simulink model "Scenario_13_CoDeSys"  (R2012b)
settings: Solver=ode3  StartTime=0.0  StopTime=inf  FixedStep=Sample_Time_Model  RelTol=1e-3
PreLoadFcn:
  | Variablen_Scenario13
InitFcn:
  | BT = randperm(9);
values from neighbouring files (symbols this model uses):
  Band_Geschwindigkeit = 1.47    [Variablen_Scenario13.m]
  Band_Sensor_Hell_2_Z = -6.5    [Variablen_Scenario13.m]
  Band_Sensor_Hell_3_Z = -10.36    [Variablen_Scenario13.m]
  Band_Sensor_Hell_4_Z = -14.64    [Variablen_Scenario13.m]
  Band_Sensor_Tolerance_Z = 0.2    [Variablen_Scenario13.m]
  Bauteil_Fallgeschwindigkeit = 0.4    [Variablen_Scenario13.m]
  Bauteil_Farbe_Metall = [0.8 0.8 0.8]    [Variablen_Scenario13.m]
  Bauteil_Farbe_Schwarz = [0.2 0.2 0.2]    [Variablen_Scenario13.m]
  Bauteil_Farbe_Weiss = [1 1 0.2]    [Variablen_Scenario13.m]
  Kran_Dauer_90_Grad = 5    [Variablen_Scenario13.m]
  Kran_Drehwinkel_90_Grad = 8050    [Variablen_Scenario13.m]
  Kran_Sensor_Position_Delta = 0.07    [Variablen_Scenario13.m]
  Sample_Time_Model = 0.05    [Variablen_Scenario13.m]
  Sample_Time_Simulation = 0.1    [Variablen_Scenario13.m]
  Sensor_Band_Metall_1 = -6.5    [Variablen_Scenario13.m]
  Sensor_Band_Metall_2 = -10.36    [Variablen_Scenario13.m]
libraries: simulink x557, vrlib x13, opclib x7, rtwinlib x1
(part 1 of 10)
settings Model: Creator=Aicher  LastModifiedBy=Aicher
settings DataIOCC: SignalLoggingSaveFormat=ModelDataLogs
settings OptimizationCC: EfficientMapNaN2IntZero=off
settings DebuggingCC: MultiTaskDSMMsg=warning  MultiTaskCondExecSysMsg=none  StrictBusMsg=None
settings HardwareCC: TargetIntDivRoundTo=Zero  TargetEndianess=LittleEndian  TargetHWDeviceType=MATLAB Host  ProdEqTarget=off
settings CodeAppCC: MaxIdLength=128
settings GRTTargetCC: CombineOutputUpdateFcns=off  GRTInterface=on

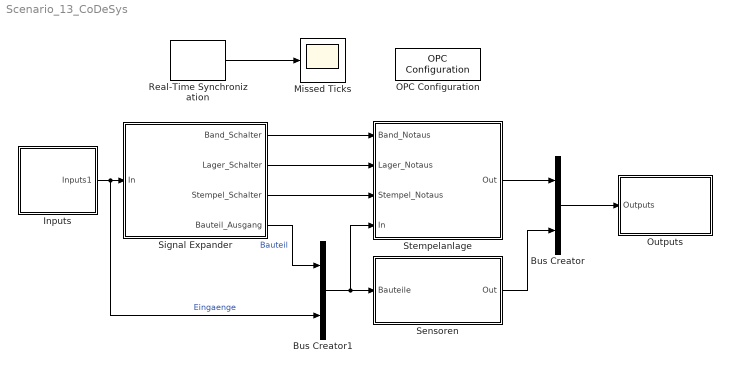
== system Scenario_13_CoDeSys ==
  Bus Creator : BusCreator  Inputs=2
  Bus Creator1 : BusCreator  Inputs=2
  Inputs : Subsystem
  Missed Ticks : Scope
      settings: TimeRange=45  YMin=0  YMax=1  DataFormat=Structure
  OPC Configuration : opclib/OPC Configuration  opcServers=localhost/CoDeSys.OPC.DA/10  errMissingItems=Error  errReadWrite=Warn  errShutdown=Error  errRTViolation=Warn  rtEnable=off  speedup=1  showLatency=off  beingUsed=on
  Outputs : Subsystem
  Real-Time Synchronization : rtwinlib/Real-Time Synchronization  SampleTime=Sample_Time_Model  MaxMissedTicks=100  ShowMissedTicks=on  YieldWhenWaiting=off
  Sensoren : Subsystem
  Signal Expander : Subsystem
  Stempelanlage : Subsystem
  wires:
  Inputs/1(Inputs1) -> Bus Creator1/2, Signal Expander/1(In)  "Eingaenge"
  Signal Expander/4(Bauteil_Ausgang) -> Bus Creator1/1  "Bauteil"
  Signal Expander/2(Lager_Schalter) -> Stempelanlage/2(Lager_Notaus)
  Stempelanlage/1(Out) -> Bus Creator/1
  Sensoren/1(Out) -> Bus Creator/2
  Bus Creator/1 -> Outputs/1(Outputs)
  Bus Creator1/1 -> Stempelanlage/4(In), Sensoren/1(Bauteile)
  Real-Time Synchronization/1 -> Missed Ticks/1
  Signal Expander/1(Band_Schalter) -> Stempelanlage/1(Band_Notaus)
  Signal Expander/3(Stempel_Schalter) -> Stempelanlage/3(Stempel_Notaus)

== system Scenario_13_CoDeSys/Inputs ==
  Bus Creator10 : BusCreator  Inputs=5
  Bus Creator11 : BusCreator  Inputs=9
  Bus Creator6 : BusCreator  Inputs=6
  Bus Creator7 : BusCreator  Inputs=6
  Bus Creator8 : BusCreator  Inputs=7
  Bus Creator9 : BusCreator  Inputs=3
  Demux2 : Demux  Outputs=19
  Demux3 : Demux  Outputs=3
  OPC Read2 : opclib/OPC Read  serverHost=localhost  serverID=CoDeSys.OPC.DA  itemIDs=PLC_GW3.Application.GVL.Stempel_Druck_Soll, PLC_GW3.Application.GVL.Stempelschlitten.QX_einfahren, PLC_GW3.Application.GVL.Stempelschlitten.QX_ausfahren, PLC_GW3.Application.GVL.Stempelzylinder.QX_einfahren, PLC_GW3.Application.GVL.Stempelzylinder.QX_ausfahren, PLC_GW3.Application.GVL.Band_vor, PLC_GW3.Application.GVL.Band_zurueck, PLC_GW3.Application.GVL.Sortierzylinder1.QX_einfahren, PLC_GW3.Application.GVL.Sortierzylinder1.QX_ausfahren, PLC_GW3.Application.GVL.Sortierzylinder2.QX_einfahren, PLC_GW3.Application.GVL.Sortierzylinder2.QX_ausfahren, PLC_GW3.Application.GVL.Vereinzelungszylinder.QX_einfahren, PLC_GW3.Application.GVL.Vereinzelungszylinder.QX_ausfahren, PLC_GW3.Application.GVL.Kran_Sauger_an, PLC_GW3.Application.GVL.Kran_Sauger_aus, PLC_GW3.Application.GVL.Kran_drehen_links, PLC_GW3.Application.GVL.Kran_drehen_rechts, PLC_GW3.Application.GVL.Kranzylinder.QX_einfahren, PLC_GW3.Application.GVL.Kranzylinder.QX_ausfahren  readMode=Asynchronous (device)  dataType=double  updateRate=Sample_Time_OPC_Fast  showQual=off  showTS=off  tsMode=Seconds since start
  OPC Read3 : opclib/OPC Read  serverHost=localhost  serverID=CoDeSys.OPC.DA  itemIDs=PLC_GW3.Application.GVL.Lager_Lampe_Gruen, PLC_GW3.Application.GVL.Band_Lampe_Gruen, PLC_GW3.Application.GVL.Stempel_Lampe_Gruen  readMode=Asynchronous (device)  dataType=double  updateRate=Sample_Time_OPC_Fast  showQual=off  showTS=off  tsMode=Seconds since start
  Rate Transition2 : RateTransition
  Rate Transition3 : RateTransition
  Subsystem1 : Subsystem
  Inputs1 : Outport
  wires:
  Demux2/15 -> Bus Creator6/2  "Kran_Sauger_Aus"
  Demux2/13 -> Bus Creator9/3  "Lager_Zyl_ausfahren"
  Demux2/12 -> Bus Creator9/2  "Lager_Zyl_einfahren"
  Demux2/11 -> Bus Creator8/7  "Band_Zyl_2_ausfahren"
  Demux2/9 -> Bus Creator8/5  "Band_Zyl_1_ausfahren"
  Demux2/10 -> Bus Creator8/6  "Band_Zyl_2_einfahren"
  Demux2/7 -> Bus Creator8/3  "Band_zurueck"
  Demux2/8 -> Bus Creator8/4  "Band_Zyl_1_einfahren"
  Demux2/5 -> Bus Creator7/6  "Stempel_ausfahren"
  Demux2/6 -> Bus Creator8/2  "Band_vor"
  Demux2/3 -> Bus Creator7/4  "Stempel_Halterung_ausfahren"
  Demux2/2 -> Bus Creator7/3  "Stempel_Halterung_einfahren"
  Demux2/4 -> Bus Creator7/5  "Stempel_einfahren"
  Bus Creator6/1 -> Bus Creator10/5  "Kran"
  Bus Creator7/1 -> Bus Creator10/2  "Stempel"
  Bus Creator8/1 -> Bus Creator10/3  "Band"
  Bus Creator9/1 -> Bus Creator10/4  "Lager"
  Bus Creator10/1 -> Inputs1/1  "Inputs"
  Subsystem1/1(BT1) -> Bus Creator11/1  "BT_Eins"
  Subsystem1/2(BT2) -> Bus Creator11/2  "BT_Zwei"
  Subsystem1/3(BT3) -> Bus Creator11/3  "BT_Drei"
  Subsystem1/4(BT4) -> Bus Creator11/4  "BT_Vier"
  Subsystem1/5(BT5) -> Bus Creator11/5  "BT_Fuenf"
  Subsystem1/6(BT6) -> Bus Creator11/6  "BT_Sechs"
  Bus Creator11/1 -> Bus Creator10/1  "Bauteile"
  OPC Read2/1 -> Rate Transition2/1
  Demux2/14 -> Bus Creator6/1  "Kran_Sauger_An"
  OPC Read3/1 -> Rate Transition3/1
  Demux2/16 -> Bus Creator6/3  "Kran_Drehen_Links"
  Demux2/17 -> Bus Creator6/4  "Kran_Drehen_Rechts"
  Demux2/18 -> Bus Creator6/5  "Kran_einfahren"
  Demux2/19 -> Bus Creator6/6  "Kran_ausfahren"
  Rate Transition3/1 -> Demux3/1
  Rate Transition2/1 -> Demux2/1
  Demux3/2 -> Bus Creator8/1  "Band_Lampe_Gruen"
  Demux2/1 -> Bus Creator7/2  "Stempel_Druck_Soll"
  Demux3/3 -> Bus Creator7/1  "Stempel_Lampe_Gruen"
  Demux3/1 -> Bus Creator9/1  "Lager_Lampe_Gruen"
  Subsystem1/7(BT7) -> Bus Creator11/7  "BT_Sieben"
  Subsystem1/8(BT8) -> Bus Creator11/8  "BT_Acht"
  Subsystem1/9(BT9) -> Bus Creator11/9  "BT_Neun"

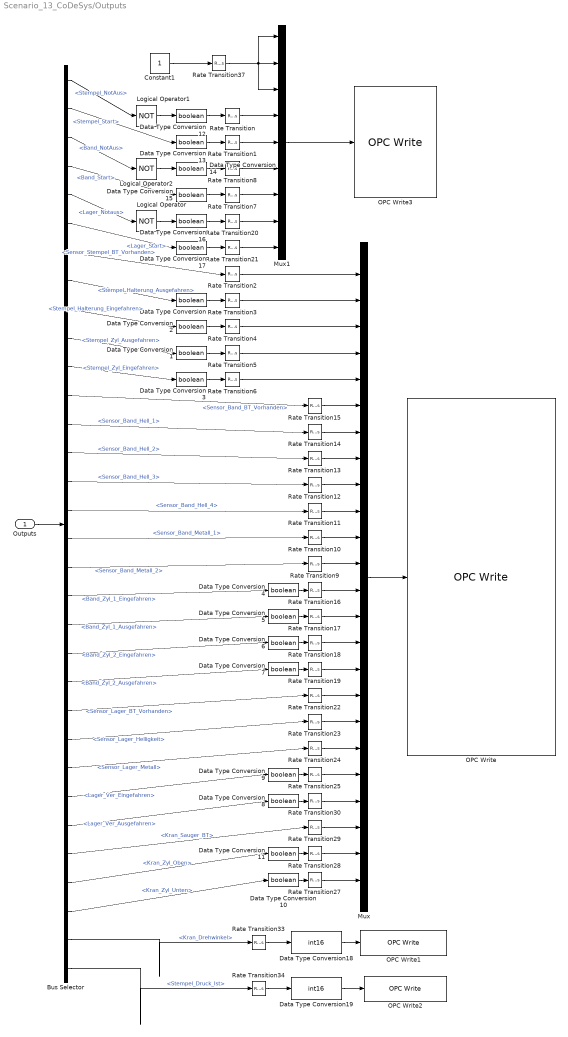
== system Scenario_13_CoDeSys/Outputs ==
  Outputs : Inport
  Bus Selector : BusSelector  OutputSignals=signal1.Stempel_Schalter.Stempel_NotAus,signal1.Stempel_Schalter.Stempel_Start,signal1.Band_Schalter.Band_NotAus,signal1.Band_Schalter.Band_Start,signal1.Lager_Schalter.Lager_Notaus,signal1.Lager_Schalter.Lager_Start,Sensoren.Sensor_Stempel_BT_Vorhanden,signal1.signal1.Bauteil.Stempelanlage_BT.Stempelanlage.Stempel.Stempel_Halterung_Ausgefahren,signal1.signal1.Bauteil.Stempelanlage_BT.Stempelanlage.Stempel.Stempel_Halterung_Eingefahren,signal1.signal1.Bauteil.Stempelanlage_BT.Stempelanlage.Stempel.Stempel_Zyl.Stempel_Zyl_Ausgefahren,signal1.signal1.Bauteil.Stempelanlage_BT.Stempelanlage.Stempel.Stempel_Zyl.Stempel_Zyl_Eingefahren,Sensoren.Sensor_Band_BT_Vorhanden,Sensoren.Sensor_Band_Hell_1,Sensoren.Sensor_Band_Hell_2,Sensoren.Sensor_Band_Hell_3,Sensoren.Sensor_Band_Hell_4,Sensoren.Sensor_Band_Metall_1,Sensoren.Sensor_Band_Metall_2,signal1.signal1.Bauteil.Stempelanlage_BT.Stempelanlage.Band.Band_Zyl_1_Eingefahren,signal1.signal1.Bauteil.Stempelanlage_BT.Stempelanlage.Band.Band_Zyl_1_Ausgefahren,signal1.signal1.Bauteil.Stempelanlage_BT.Stempelanlage.Band.Band_Zyl_2_Eingefahren,signal1.signal1.Bauteil.Stempelanlage_BT.Stempelanlage.Band.Band_Zyl_2_Ausgefahren,Sensoren.Sensor_Lager_BT_Vorhanden,Sensoren.Sensor_Lager_Helligkeit,Sensoren.Sensor_Lager_Metall,signal1.signal1.Bauteil.Stempelanlage_BT.Stempelanlage.Lager.Lager_Ver_Eingefahren,signal1.signal1.Bauteil.Stempelanlage_BT.Stempelanlage.Lager.Lager_Ver_Ausgefahren,Sensoren.Kran_Sauger_BT,signal1.signal1.Bauteil.Stempelanlage_BT.Stempelanlage.Kran.Kran_Zyl.Kran_Zyl_Oben,signal1.signal1.Bauteil.Stempelanlage_BT.Stempelanlage.Kran.Kran_Zyl.Kran_Zyl_Unten,signal1.signal1.Bauteil.Stempelanlage_BT.Stempelanlage.Kran.Kran_Drehwinkel,Sensoren.Stempel_Druck_Ist
  Constant1 : Constant  OutDataTypeStr=boolean
  Data Type Conversion{,1..17} (18 alike) : DataTypeConversion  OutDataTypeStr=boolean
  Data Type Conversion18 : DataTypeConversion  OutDataTypeStr=int16
  Data Type Conversion19 : DataTypeConversion  OutDataTypeStr=int16
  Logical Operator : Logic  Operator=NOT  AllPortsSameDT=off  OutDataTypeStr=boolean
  Logical Operator1 : Logic  Operator=NOT  AllPortsSameDT=off
  Logical Operator2 : Logic  Operator=NOT  AllPortsSameDT=off  OutDataTypeStr=boolean
  Mux : Mux  Inputs=24
  Mux1 : Mux  Inputs=9
  OPC Write : opclib/OPC Write  serverHost=localhost  serverID=CoDeSys.OPC.DA  itemIDs=PLC_GW3.Application.GVL.Stempel_Sensor_Mat_vorhanden, PLC_GW3.Application.GVL.Stempelschlitten.IX_ausgefahren, PLC_GW3.Application.GVL.Stempelschlitten.IX_eingefahren, PLC_GW3.Application.GVL.Stempelzylinder.IX_ausgefahren, PLC_GW3.Application.GVL.Stempelzylinder.IX_eingefahren, PLC_GW3.Application.GVL.Band_Sensor_Mat_Vorhanden, PLC_GW3.Application.GVL.Band_Sensor_Hell_1, PLC_GW3.Application.GVL.Band_Sensor_Hell_2, PLC_GW3.Application.GVL.Band_Sensor_Hell_3, PLC_GW3.Application.GVL.Band_Sensor_Hell_4, PLC_GW3.Application.GVL.Band_Sensor_Metall_1, PLC_GW3.Application.GVL.Band_Sensor_Metall_2, PLC_GW3.Application.GVL.Sortierzylinder1.IX_eingefahren, PLC_GW3.Application.GVL.Sortierzylinder1.IX_ausgefahren, PLC_GW3.Application.GVL.Sortierzylinder2.IX_eingefahren, PLC_GW3.Application.GVL.Sortierzylinder2.IX_ausgefahren, PLC_GW3.Application.GVL.Lager_Sensor_Mat_Vorhanden, PLC_GW3.Application.GVL.Lager_Sensor_Hell, PLC_GW3.Application.GVL.Lager_Sensor_Metall, PLC_GW3.Application.GVL.Vereinzelungszylinder.IX_eingefahren, PLC_GW3.Application.GVL.Vereinzelungszylinder.IX_ausgefahren, PLC_GW3.Application.GVL.Kran_Mat_angesaugt, PLC_GW3.Application.GVL.Kranzylinder.IX_ausgefahren, PLC_GW3.Application.GVL.Kranzylinder.IX_eingefahren  writeMode=Asynchronous  updateRate=0.1
  OPC Write1 : opclib/OPC Write  serverHost=localhost  serverID=CoDeSys.OPC.DA  itemIDs=PLC_GW3.Application.GVL.Kran_Drehwinkel  writeMode=Asynchronous  updateRate=0.05
  OPC Write2 : opclib/OPC Write  serverHost=localhost  serverID=CoDeSys.OPC.DA  itemIDs=PLC_GW3.Application.GVL.Stempel_Druck_Ist  writeMode=Asynchronous  updateRate=0.1
  OPC Write3 : opclib/OPC Write  serverHost=localhost  serverID=CoDeSys.OPC.DA  itemIDs=PLC_GW3.Application.GVL.Stempel_Man_Auto, PLC_GW3.Application.GVL.Band_Man_Auto, PLC_GW3.Application.GVL.Lager_Man_Auto, PLC_GW3.Application.GVL.Nicht_Notaus_Stempel, PLC_GW3.Application.GVL.Stempel_Start, PLC_GW3.Application.GVL.Nicht_Notaus_Band, PLC_GW3.Application.GVL.Band_Start, PLC_GW3.Application.GVL.Nicht_Notaus_Lager, PLC_GW3.Application.GVL.Lager_Start  writeMode=Asynchronous  updateRate=0.1
  Rate Transition{,1..25,27..30,33..34,37} (33 alike) : RateTransition
  wires:
  Outputs/1 -> Bus Selector/1
  Bus Selector/30 -> Data Type Conversion10/1  "<Kran_Zyl_Unten>"
  Bus Selector/5 -> Logical Operator/1  "<Lager_Notaus>"
  Bus Selector/19 -> Data Type Conversion4/1  "<Band_Zyl_1_Eingefahren>"
  Bus Selector/8 -> Data Type Conversion/1  "<Stempel_Halterung_Ausgefahren>"
  Bus Selector/11 -> Data Type Conversion3/1  "<Stempel_Zyl_Eingefahren>"
  Bus Selector/23 -> Rate Transition22/1  "<Sensor_Lager_BT_Vorhanden>"
  Bus Selector/1 -> Logical Operator1/1  "<Stempel_NotAus>"
  Bus Selector/21 -> Data Type Conversion6/1  "<Band_Zyl_2_Eingefahren>"
  Bus Selector/3 -> Logical Operator2/1  "<Band_NotAus>"
  Bus Selector/9 -> Data Type Conversion2/1  "<Stempel_Halterung_Eingefahren>"
  Bus Selector/6 -> Data Type Conversion17/1  "<Lager_Start>"
  Bus Selector/7 -> Rate Transition2/1  "<Sensor_Stempel_BT_Vorhanden>"
  Bus Selector/22 -> Data Type Conversion7/1  "<Band_Zyl_2_Ausgefahren>"
  Bus Selector/10 -> Data Type Conversion1/1  "<Stempel_Zyl_Ausgefahren>"
  Bus Selector/20 -> Data Type Conversion5/1  "<Band_Zyl_1_Ausgefahren>"
  Bus Selector/2 -> Data Type Conversion13/1  "<Stempel_Start>"
  Bus Selector/24 -> Rate Transition23/1  "<Sensor_Lager_Helligkeit>"
  Bus Selector/27 -> Data Type Conversion8/1  "<Lager_Ver_Ausgefahren>"
  Bus Selector/25 -> Rate Transition24/1  "<Sensor_Lager_Metall>"
  Bus Selector/26 -> Data Type Conversion9/1  "<Lager_Ver_Eingefahren>"
  Bus Selector/29 -> Data Type Conversion11/1  "<Kran_Zyl_Oben>"
  Bus Selector/28 -> Rate Transition29/1  "<Kran_Sauger_BT>"
  Mux/1 -> OPC Write/1
  Data Type Conversion/1 -> Rate Transition3/1
  Data Type Conversion2/1 -> Rate Transition4/1
  Data Type Conversion1/1 -> Rate Transition5/1
  Data Type Conversion3/1 -> Rate Transition6/1
  Data Type Conversion4/1 -> Rate Transition16/1
  Data Type Conversion5/1 -> Rate Transition17/1
  Data Type Conversion7/1 -> Rate Transition19/1
  Data Type Conversion9/1 -> Rate Transition25/1
  Data Type Conversion8/1 -> Rate Transition30/1
  Data Type Conversion11/1 -> Rate Transition28/1
  Data Type Conversion10/1 -> Rate Transition27/1
  Bus Selector/31 -> Rate Transition33/1  "<Kran_Drehwinkel>"
  Bus Selector/4 -> Data Type Conversion15/1  "<Band_Start>"
  Bus Selector/32 -> Rate Transition34/1  "<Stempel_Druck_Ist>"
  Data Type Conversion6/1 -> Rate Transition18/1
  Logical Operator/1 -> Data Type Conversion16/1
  Logical Operator1/1 -> Data Type Conversion12/1
  Logical Operator2/1 -> Data Type Conversion14/1
  Constant1/1 -> Rate Transition37/1
  Mux1/1 -> OPC Write3/1
  Rate Transition/1 -> Mux1/4
  Rate Transition1/1 -> Mux1/5
  Rate Transition2/1 -> Mux/1
  Rate Transition3/1 -> Mux/2
  Rate Transition4/1 -> Mux/3
  Rate Transition5/1 -> Mux/4
  Rate Transition6/1 -> Mux/5
  Rate Transition8/1 -> Mux1/6
  Rate Transition7/1 -> Mux1/7
  Rate Transition16/1 -> Mux/13
  Rate Transition17/1 -> Mux/14
  Rate Transition18/1 -> Mux/15
  Rate Transition19/1 -> Mux/16
  Rate Transition20/1 -> Mux1/8
  Rate Transition21/1 -> Mux1/9
  Rate Transition22/1 -> Mux/17
  Rate Transition23/1 -> Mux/18
  Rate Transition24/1 -> Mux/19
  Rate Transition25/1 -> Mux/20
  Rate Transition30/1 -> Mux/21
  Rate Transition29/1 -> Mux/22
  Rate Transition28/1 -> Mux/23
  Rate Transition27/1 -> Mux/24
  Rate Transition33/1 -> Data Type Conversion18/1
  Rate Transition34/1 -> Data Type Conversion19/1
  Rate Transition37/1 -> Mux1/3, Mux1/1, Mux1/2
  Data Type Conversion12/1 -> Rate Transition/1
  Data Type Conversion17/1 -> Rate Transition21/1
  Data Type Conversion16/1 -> Rate Transition20/1
  Data Type Conversion15/1 -> Rate Transition7/1
  Data Type Conversion14/1 -> Rate Transition8/1
  Data Type Conversion13/1 -> Rate Transition1/1
  Bus Selector/13 -> Rate Transition14/1  "<Sensor_Band_Hell_1>"
  Bus Selector/18 -> Rate Transition9/1  "<Sensor_Band_Metall_2>"
  Bus Selector/17 -> Rate Transition10/1  "<Sensor_Band_Metall_1>"
  Bus Selector/16 -> Rate Transition11/1  "<Sensor_Band_Hell_4>"
  Bus Selector/15 -> Rate Transition12/1  "<Sensor_Band_Hell_3>"
  Bus Selector/14 -> Rate Transition13/1  "<Sensor_Band_Hell_2>"
  Bus Selector/12 -> Rate Transition15/1  "<Sensor_Band_BT_Vorhanden>"
  Rate Transition9/1 -> Mux/12
  Rate Transition10/1 -> Mux/11
  Rate Transition11/1 -> Mux/10
  Rate Transition12/1 -> Mux/9
  Rate Transition13/1 -> Mux/8
  Rate Transition14/1 -> Mux/7
  Rate Transition15/1 -> Mux/6
  Data Type Conversion18/1 -> OPC Write1/1
  Data Type Conversion19/1 -> OPC Write2/1

== system Scenario_13_CoDeSys/Sensoren ==
  Bauteile : Inport
  Bus Creator1 : BusCreator  Inputs=13
  Bus Selector4 : BusSelector  OutputSignals=Bauteil.Stempelanlage_BT.Bauteil_1.Kran_Sauger_BT_1,Bauteil.Stempelanlage_BT.Bauteil_2.Kran_Sauger_BT_2,Bauteil.Stempelanlage_BT.Bauteil_3.Kran_Sauger_BT_3,Bauteil.Stempelanlage_BT.Bauteil_4.Kran_Sauger_BT_4,Bauteil.Stempelanlage_BT.Bauteil_5.Kran_Sauger_BT_5,Bauteil.Stempelanlage_BT.Bauteil_6.Kran_Sauger_BT_6,Bauteil.Stempelanlage_BT.Bauteil_7.Kran_Sauger_BT_7,Bauteil.Stempelanlage_BT.Bauteil_8.Kran_Sauger_BT_8,Bauteil.Stempelanlage_BT.Bauteil_9.Kran_Sauger_BT_9
  Bus Selector5 : BusSelector  OutputSignals=Bauteil.Stempelanlage_BT.Stempelanlage.Stempel.Stempel_Halterung_Eingefahren,Bauteil.Stempelanlage_BT.Stempelanlage.Stempel.Stempel_Zyl.Stempel_Zyl_Ausgefahren
  Bus Selector6 : BusSelector  OutputSignals=Eingaenge.Stempel.Stempel_Druck_Soll
  Display{,1..12} (13 alike) : Display
  Kran_Sauger_BT : Subsystem
  Sensor_Band_BT_Vorhanden_Hell_1 : Subsystem
  Sensor_Band_Hell_2 : Subsystem
  Sensor_Band_Hell_3 : Subsystem
  Sensor_Band_Hell_4 : Subsystem
  Sensor_Band_Metall_1 : Subsystem
  Sensor_Band_Metall_2 : Subsystem
  Sensor_Lager_BT_Vorhanden : Subsystem
  Sensor_Stempel_BT_Vorhanden : Subsystem
  Sensoren_Lager_Metall_und_Weiss_Schwarz : Subsystem
  Stempel_Druck_Ist : Subsystem
  Out : Outport
  wires:
  Bus Selector4/1 -> Kran_Sauger_BT/1(BT_1)  "<Kran_Sauger_BT_1>"
  Bus Selector4/2 -> Kran_Sauger_BT/2(BT_2)  "<Kran_Sauger_BT_2>"
  Sensor_Stempel_BT_Vorhanden/1(Sensor_Stempel_BT_Vorhanden) -> Stempel_Druck_Ist/1(Sensor_Stempel_BT_Vorhanden), Display/1, Bus Creator1/5  "Sensor_Stempel_BT_Vorhanden"
  Kran_Sauger_BT/1(Kran_Sauger_BT) -> Display1/1, Bus Creator1/4  "Kran_Sauger_BT"
  Sensor_Lager_BT_Vorhanden/1(Sensor_Lager_BT_Vorhanden) -> Display2/1, Bus Creator1/3  "Sensor_Lager_BT_Vorhanden"
  Bus Creator1/1 -> Out/1  "Sensoren"
  Bus Selector5/1 -> Stempel_Druck_Ist/2(Stempel_Halterung_Eingefahren)  "<Stempel_Halterung_Eingefahren>"
  Bus Selector5/2 -> Stempel_Druck_Ist/3(Stempel_Zyl_Ausgefahren)  "<Stempel_Zyl_Ausgefahren>"
  Stempel_Druck_Ist/1(Stempel_Druck_Ist) -> Display5/1, Bus Creator1/6  "Stempel_Druck_Ist"
  Bus Selector6/1 -> Stempel_Druck_Ist/4(Stempel_Druck_Soll)  "<Stempel_Druck_Soll>"
  Sensoren_Lager_Metall_und_Weiss_Schwarz/1(Sensor_Lager_Metall) -> Display4/1, Bus Creator1/1  "Sensor_Lager_Metall"
  Sensoren_Lager_Metall_und_Weiss_Schwarz/2(Sensor_Lager_Helligkeit) -> Display3/1, Bus Creator1/2  "Sensor_Lager_Helligkeit"
  Bauteile/1 -> Sensoren_Lager_Metall_und_Weiss_Schwarz/1(In), Sensor_Lager_BT_Vorhanden/1(In), Sensor_Band_Hell_4/1(Inputs), Sensor_Band_Metall_2/1(Inputs), Sensor_Band_Metall_1/1(Inputs), Sensor_Band_Hell_3/1(Inputs), Sensor_Band_Hell_2/1(Inputs), Sensor_Band_BT_Vorhanden_Hell_1/1(Inputs), Bus Selector6/1, Bus Selector5/1, Sensor_Stempel_BT_Vorhanden/1(In), Bus Selector4/1
  Bus Selector4/3 -> Kran_Sauger_BT/3(BT_3)  "<Kran_Sauger_BT_3>"
  Bus Selector4/6 -> Kran_Sauger_BT/6(BT_6)  "<Kran_Sauger_BT_6>"
  Bus Selector4/5 -> Kran_Sauger_BT/5(BT_5)  "<Kran_Sauger_BT_5>"
  Bus Selector4/4 -> Kran_Sauger_BT/4(BT_4)  "<Kran_Sauger_BT_4>"
  Bus Selector4/7 -> Kran_Sauger_BT/7(BT_7)  "<Kran_Sauger_BT_7>"
  Bus Selector4/9 -> Kran_Sauger_BT/9(BT_9)  "<Kran_Sauger_BT_9>"
  Bus Selector4/8 -> Kran_Sauger_BT/8(BT_8)  "<Kran_Sauger_BT_8>"
  Sensor_Band_BT_Vorhanden_Hell_1/1(Sensor_Band_BT_Vorhanden) -> Display6/1, Bus Creator1/7  "Sensor_Band_BT_Vorhanden"
  Sensor_Band_BT_Vorhanden_Hell_1/2(Sensor_Band_Hell_1) -> Display7/1, Bus Creator1/8  "Sensor_Band_Hell_1"
  Sensor_Band_Hell_2/1(Sensor_Band_Hell_2) -> Display8/1, Bus Creator1/9  "Sensor_Band_Hell_2"
  Sensor_Band_Hell_4/1(Sensor_Band_Hell_4) -> Display10/1, Bus Creator1/11  "Sensor_Band_Hell_4"
  Sensor_Band_Metall_1/1(Sensor_Band_Metall_1) -> Display11/1, Bus Creator1/12  "Sensor_Band_Metall_1"
  Sensor_Band_Metall_2/1(Sensor_Band_Metall_2) -> Bus Creator1/13, Display12/1  "Sensor_Band_Metall_2"
  Sensor_Band_Hell_3/1(Sensor_Band_Hell_3) -> Display9/1, Bus Creator1/10  "Sensor_Band_Hell_3"

== stateflow chart Scenario_13_CoDeSys/Signal Expander/Bauteil_7 ==
  state Bauteil_Pos_7
    entry:
    BT_X_Achse = 5.75;
    BT_Y_Achse = 6.84;
    x =0;
  state Bauteil_Faellt3
    during:
    BT_Y_Achse = Next_Pos_Minus_Min(BT_Y_Achse, Bauteil_Fallgeschwindigkeit, 5.83);
  state Bauteil_Pos_6
    entry:
    BT_X_Achse = 5.75;
    BT_Y_Achse = 5.81;
    x =0;
  state Bauteil_Faellt2
    during:
    BT_Y_Achse = Next_Pos_Minus_Min(BT_Y_Achse, Bauteil_Fallgeschwindigkeit, 4.8);
  state Stop1
  state Bauteil_Pos_2
  state Bauteil_Unten
  state Bauteil_Pos_5
  state Bauteil_Faellt_3
    during:
    BT_Y_Achse = Next_Pos_Minus_Min(BT_Y_Achse, Bauteil_Fallgeschwindigkeit, 0.7);
  state Drehen_Rechts_Runter [function]
    (default) -> (junction 322) : {BT_Y_Achse = Next_Pos_Minus_Min(BT_Y_Achse, Kran_Zyl_Schritt_Runter, 0.65);
        | x = x - Kran_Drehen_Schritt;
        | BT_Z_Achse = -3.5*sin(x);
        | BT_X_Achse = 3.5*cos(x);}
  state Bauteil_Faellt1
    during:
    BT_Y_Achse = Next_Pos_Minus_Min(BT_Y_Achse, Bauteil_Fallgeschwindigkeit, 3.77);
  state Drehen_Rechts_Hoch [function]
    (default) -> (junction 325) : {BT_Y_Achse = Next_Pos_Plus_Max(BT_Y_Achse, Kran_Zyl_Schritt_Hoch, 1.65);
        | x = x - Kran_Drehen_Schritt;
        | BT_Z_Achse = -3.5*sin(x);
        | BT_X_Achse = 3.5*cos(x);}
  state Bauteil_Lager_Vereinz_Ausfahren
    during:
    BT_X_Achse = BT_X_Achse - Lager_Vereinzler_Schritt_Aus;
  state Bauteil_Lager_Bereit
    entry: BT_Bereit = 1;
    BT_X_Achse = 3.5;
  state Drehen_Links_Runter [function]
    (default) -> (junction 319) : {BT_Y_Achse = Next_Pos_Minus_Min(BT_Y_Achse, Kran_Zyl_Schritt_Runter, 0.65);
        | x = x + Kran_Drehen_Schritt;
        | BT_Z_Achse = -3.5*sin(x);
        | BT_X_Achse = 3.5*cos(x);}
  state Drehen_Links_Hoch [function]
    (default) -> (junction 309) : {BT_Y_Achse = Next_Pos_Plus_Max(BT_Y_Achse, Kran_Zyl_Schritt_Hoch, 1.65);
        | x = x + Kran_Drehen_Schritt;
        | BT_Z_Achse = -3.5*sin(x);
        | BT_X_Achse = 3.5*cos(x);}
  state Ausgabe = Next_Pos_Plus_Max(Achse, Schrittgroesse, MaxWert) [function]
    (default) -> (junction 249) : {Naechste_Position = Achse + Schrittgroesse;}
    (junction 249) -> (junction 250) [order 1] : [Naechste_Position >= MaxWert]
    (junction 249) -> (junction 251) [order 2] : {Ausgabe = Naechste_Position;}
    (junction 250) -> (junction 252) : {Ausgabe = MaxWert;}
    (junction 252) -> (junction 251)
  state Bauteil_Pos_3
  state Bauteil_Kran_Hochheben_Bereit
    entry: BT_Bereit = 1;
    Kran_Sauger_BT = 1;
  state Bauteil_Faellt_2
    during:
    BT_Y_Achse = Next_Pos_Minus_Min(BT_Y_Achse, Bauteil_Fallgeschwindigkeit, 1.73);
  state Bauteil_Pos_4
  state Bauteil_Faellt
    during:
    BT_Y_Achse = Next_Pos_Minus_Min(BT_Y_Achse, Bauteil_Fallgeschwindigkeit, 2.75);
  state Ausgabe = Next_Pos_Minus_Min(Achse, Schrittgroesse, MinWert) [function]
    (default) -> (junction 268) : {Naechste_Position = Achse - Schrittgroesse;}
    (junction 268) -> (junction 269) [order 1] : [Naechste_Position <= MinWert]
    (junction 268) -> (junction 270) [order 2] : {Ausgabe = Naechste_Position;}
    (junction 269) -> (junction 271) : {Ausgabe = MinWert;}
    (junction 271) -> (junction 270)
  state Ausgabe = Lager_Y_Achse(Lager_Status, Pos_1, Pos_2, Pos_3) [function]
    (default) -> (junction 398)
    (junction 398) -> (junction 397) [order 3] : [Lager_Status == 2]
    (junction 398) -> (junction 399) [order 1] : [Lager_Status == 0]
    (junction 397) -> (junction 400) : {Ausgabe = Pos_3;}
    (junction 398) -> (junction 401) [order 2] : [Lager_Status == 1]
        | {Ausgabe = Pos_2;}
    (junction 399) -> (junction 402) : {Ausgabe = Pos_1;}
    (junction 400) -> (junction 401)
    (junction 402) -> (junction 401)
  state Bauteil_Stempel_Halterung_Einfahren
    during:
    BT_X_Achse = Next_Pos_Minus_Min(BT_X_Achse, Stempel_Halterung_Schritt_Ein, -4.6);
  state Bauteil_Kran_Runterlassen
    during:
    BT_Y_Achse = Next_Pos_Minus_Min(BT_Y_Achse, Kran_Zyl_Schritt_Runter, 0.65);
  state Bauteil_Kran_Hochheben
    during:
    BT_Y_Achse = Next_Pos_Plus_Max(BT_Y_Achse, Kran_Zyl_Schritt_Hoch, 1.65);
  state Bauteil_Faellt_Auf_Festen_Untergrund
  state Bauteil_Lost
  state Bauteil_Lager_1_Ende
    entry: BT_Y_Achse = Lager_Y_Achse(Lager_1_Status, -0.158, 0.037, 0.232);
    BT_Lager = 1;
  state Bauteil_Abgesetzt_Stempel
    entry: Kran_Sauger_BT = 0;
  state Bauteil_Kran_Zyl_Stop
  state Bauteil_Stempel_Halterung_Stop
  state Drop_Down
    entry: Kran_Sauger_BT = 0;
    during:
    BT_Y_Achse = BT_Y_Achse - 0.4;
  state Bauteil_Lager_1_Beginnt
    entry: BT_Rotation_1 = 0;
    BT_Rotation_2 = 0;
    BT_Rotation_3 = 1;
    BT_Rotation_4 = 0.2;
    during:
    BT_X_Achse = Next_Pos_Minus_Min(BT_X_Achse, Band_Zyl_1_Schritt, -6.5 + Lager_1_Status);
    BT_Y_Achse = BT_Y_Achse - (0.2 * Band_Zyl_1_Schritt);
  state Bauteil_Stempel_Halterung_Ausfahren
    during:
    BT_X_Achse = Next_Pos_Plus_Max(BT_X_Achse, Stempel_Halterung_Schritt_Aus, -3.4);
  note: Bei -2,8 beginnt in etwa die Schraege !!
  state Drehen_Links
    during:
    x = x + Kran_Drehen_Schritt;
    BT_Z_Achse = -3.5*sin(x);
    BT_X_Achse = 3.5*cos(x);
  state Bauteil_Band_Vor
    during:
    BT_Z_Achse = BT_Z_Achse - Band_Geschwindigkeit;
  state Bauteil_Lager_1_Schieben
    during:
    BT_X_Achse = Next_Pos_Minus_Min(BT_X_Achse, Band_Zyl_1_Schritt, -2.7);
  state Bauteil_Lager_2_Ende
    entry: BT_Y_Achse = Lager_Y_Achse(Lager_2_Status, -0.158, 0.037, 0.232);
    BT_Lager = 2;
  state Bauteil_Kran_Rot_Stop
  state Bauteil_Band_Stop
    entry: Kran_Sauger_BT = 0;
  state Drehen_Rechts
    during:
    x = x - Kran_Drehen_Schritt;
    BT_Z_Achse = -3.5*sin(x);
    BT_X_Achse = 3.5*cos(x);
  state Bauteil_Lager_2_Beginnt
    entry: BT_Rotation_1 = 0;
    BT_Rotation_2 = 0;
    BT_Rotation_3 = 1;
    BT_Rotation_4 = 0.2;
    during:
    BT_X_Achse = Next_Pos_Minus_Min(BT_X_Achse, Band_Zyl_2_Schritt, -6.5 + Lager_2_Status);
    BT_Y_Achse = BT_Y_Achse - (0.2 * Band_Zyl_2_Schritt);
  state Bauteil_Band_Zurueck
    during:
    BT_Z_Achse = BT_Z_Achse + Band_Geschwindigkeit;
  state Bauteil_Lager_2_Schieben
    during:
    BT_X_Achse = Next_Pos_Minus_Min(BT_X_Achse, Band_Zyl_2_Schritt, -2.7);
  state Bauteil_Kran_Runterlassen_Und_Drehen_Rechts
    entry:
    x = x - Kran_Drehen_Schritt;
    BT_Z_Achse = -3.5*sin(x);
    BT_X_Achse = 3.5*cos(x);
    during: Drehen_Rechts_Runter();
  state Bauteil_Lager_3_Beginnt
    entry: BT_Rotation_1 = -1;
    BT_Rotation_2 = 0;
    BT_Rotation_3 = 0;
    BT_Rotation_4 = 0.2;
    during:
    BT_Z_Achse = Next_Pos_Minus_Min(BT_Z_Achse, 1.5 * Band_Geschwindigkeit, -19.05 + Lager_3_Status);
    BT_Y_Achse = BT_Y_Achse - (1.5 * 0.2*Band_Geschwindigkeit);
  state Bauteil_Kran_Hochheben_Und_Drehen_Links
    entry:
    x = x + Kran_Drehen_Schritt;
    BT_Z_Achse = -3.5*sin(x);
    BT_X_Achse = 3.5*cos(x);
    during: Drehen_Links_Hoch();
  state Bauteil_Lager_3_Ende
    entry: BT_Y_Achse = Lager_Y_Achse(Lager_3_Status, -0.158, 0.037, 0.232);
    BT_Lager = 3;
  state Bauteil_Kran_Hochheben_Und_Drehen_Rechts
    entry:
    x = x - Kran_Drehen_Schritt;
    BT_Z_Achse = -3.5*sin(x);
    BT_X_Achse = 3.5*cos(x);
    during:Drehen_Rechts_Hoch();
  state Bauteil_Kran_Runterlassen_Und_Drehen_Links
    entry:
    x = x + Kran_Drehen_Schritt;
    BT_Z_Achse = -3.5*sin(x);
    BT_X_Achse = 3.5*cos(x);
    during: Drehen_Links_Runter();
  (default) -> Bauteil_Pos_7
  Bauteil_Faellt_Auf_Festen_Untergrund -> Bauteil_Abgesetzt_Stempel [order 2] : [Kran_Stellung_Stempel]
  Bauteil_Pos_7 -> Bauteil_Faellt3 : [BT_1_Bereit && Lager_Ver_Eingefahren]
  Bauteil_Faellt3 -> Bauteil_Pos_6 : [BT_Y_Achse <= 5.83]
  Bauteil_Pos_6 -> Bauteil_Faellt2 : [BT_2_Bereit && Lager_Ver_Eingefahren]
  Bauteil_Faellt2 -> Bauteil_Pos_5 : [BT_Y_Achse <= 4.8]
  Stop1 -> Bauteil_Lager_Vereinz_Ausfahren : [BT_X_Achse + Lager_X_Achse >= 5.1]
  Bauteil_Lager_Vereinz_Ausfahren -> Stop1 [order 2] : [BT_X_Achse + Lager_X_Achse < 5.1]
  Bauteil_Pos_2 -> Bauteil_Faellt_3 : [BT_6_Bereit && Lager_Ver_Eingefahren]
  Bauteil_Unten -> Bauteil_Lager_Vereinz_Ausfahren : [Lager_Ver_Ausfahren && (BT_X_Achse + Lager_X_Achse >= 5.1)]
  Bauteil_Pos_5 -> Bauteil_Faellt1 : [BT_3_Bereit && Lager_Ver_Eingefahren]
  Bauteil_Faellt_2 -> Bauteil_Pos_2 : [BT_Y_Achse <= 1.73]
  Bauteil_Faellt_3 -> Bauteil_Unten : [BT_Y_Achse <= 0.7]
  Bauteil_Lager_Vereinz_Ausfahren -> Bauteil_Lager_Bereit [order 1] : [Lager_Ver_Ausgefahren]
  Bauteil_Faellt1 -> Bauteil_Pos_4 : [BT_Y_Achse <= 3.77]
  Bauteil_Faellt_Auf_Festen_Untergrund -> Bauteil_Lager_Bereit [order 1] : [Kran_Stellung_Lager]
  Bauteil_Lager_Bereit -> Bauteil_Kran_Hochheben_Bereit : [Kran_Stellung_Lager && Kran_Sauger && Kran_Zyl_Unten]
  Bauteil_Stempel_Halterung_Stop -> Bauteil_Kran_Hochheben_Bereit [order 3] : [Kran_Stellung_Stempel && Kran_Sauger && Kran_Zyl_Unten]
  (junction 127) -> Bauteil_Kran_Hochheben_Bereit [order 2] : [Kran_Stellung_Lager && Kran_Sauger && Kran_Zyl_Unten]
  Bauteil_Faellt -> Bauteil_Pos_3 : [BT_Y_Achse <= 2.75]
  Bauteil_Kran_Hochheben_Bereit -> Bauteil_Kran_Hochheben : [Kran_Hochheben]
      | {BT_Bereit = 0;}
  Bauteil_Pos_3 -> Bauteil_Faellt_2 : [BT_5_Bereit && Lager_Ver_Eingefahren]
  Bauteil_Pos_4 -> Bauteil_Faellt : [BT_4_Bereit && Lager_Ver_Eingefahren]
  Bauteil_Kran_Hochheben -> (junction 127) [order 3]
  Bauteil_Kran_Rot_Stop -> (junction 287) [order 4]
  (junction 287) -> Bauteil_Kran_Hochheben [order 2] : [Kran_Hochheben]
  (junction 287) -> Bauteil_Kran_Runterlassen [order 1] : [Kran_Runterlassen]
  Bauteil_Stempel_Halterung_Stop -> Bauteil_Stempel_Halterung_Einfahren [order 1] : [Stempel_Halterung_Einfahren]
  Bauteil_Stempel_Halterung_Einfahren -> Bauteil_Stempel_Halterung_Stop : [!Stempel_Halterung_Einfahren]
  Bauteil_Kran_Hochheben -> Bauteil_Kran_Runterlassen [order 1] : [Kran_Runterlassen]
  Bauteil_Kran_Runterlassen -> (junction 127) [order 2]
  Bauteil_Kran_Runterlassen -> (junction 162) [order 4]
  Bauteil_Kran_Zyl_Stop -> Bauteil_Kran_Runterlassen [order 3] : [Kran_Runterlassen]
  Bauteil_Kran_Runterlassen -> Bauteil_Kran_Zyl_Stop [order 3] : [Kran_Zyl_Unten]
  Bauteil_Kran_Runterlassen -> Bauteil_Kran_Hochheben [order 1] : [Kran_Hochheben]
  Drop_Down -> Bauteil_Faellt_Auf_Festen_Untergrund [order 2] : [(Kran_Stellung_Band || Kran_Stellung_Lager || Kran_Stellung_Stempel) && (BT_Y_Achse <= 0.65)]
  Drop_Down -> Bauteil_Lost [order 1] : [BT_Y_Achse <= -2]
  Bauteil_Kran_Hochheben -> (junction 162) [order 4]
  Bauteil_Kran_Hochheben -> Bauteil_Kran_Zyl_Stop [order 2] : [Kran_Zyl_Oben]
  Bauteil_Kran_Zyl_Stop -> Bauteil_Kran_Hochheben [order 2] : [Kran_Hochheben]
  Bauteil_Lager_1_Beginnt -> Bauteil_Lager_1_Ende : [BT_X_Achse <= (-6.5 + Lager_1_Status)]
  Bauteil_Abgesetzt_Stempel -> Bauteil_Stempel_Halterung_Stop
  Bauteil_Faellt_Auf_Festen_Untergrund -> Bauteil_Band_Stop [order 3] : [Kran_Stellung_Band]
  (junction 127) -> Drop_Down [order 1] : [!Kran_Sauger]
  Bauteil_Kran_Zyl_Stop -> (junction 127) [order 8]
  Bauteil_Kran_Zyl_Stop -> Bauteil_Abgesetzt_Stempel [order 6] : [Kran_Zyl_Unten && !Kran_Sauger && Kran_Stellung_Stempel]
  Drehen_Rechts -> Drop_Down [order 3] : [!Kran_Sauger]
  Bauteil_Stempel_Halterung_Ausfahren -> Bauteil_Stempel_Halterung_Stop : [!Stempel_Halterung_Ausfahren]
  Bauteil_Stempel_Halterung_Stop -> Bauteil_Stempel_Halterung_Ausfahren [order 2] : [Stempel_Halterung_Ausfahren]
  Bauteil_Kran_Rot_Stop -> Drop_Down [order 3] : [!Kran_Sauger]
  Drehen_Links -> Drop_Down [order 3] : [!Kran_Sauger]
  Bauteil_Kran_Zyl_Stop -> Drehen_Links [order 4] : [Kran_Drehen_Links]
  Bauteil_Kran_Zyl_Stop -> Drehen_Rechts [order 5] : [Kran_Drehen_Rechts]
  (junction 178) -> Bauteil_Kran_Zyl_Stop : [!Kran_Drehen_Rechts && !Kran_Drehen_Links]
  Bauteil_Kran_Zyl_Stop -> (junction 162) [order 1]
  Bauteil_Kran_Zyl_Stop -> Bauteil_Band_Stop [order 7] : [Kran_Zyl_Unten && !Kran_Sauger && Kran_Stellung_Band]
  Bauteil_Band_Stop -> Bauteil_Kran_Zyl_Stop [order 3] : [Kran_Zyl_Unten && Kran_Sauger && Kran_Stellung_Band && (-3.8 <= BT_Z_Achse) && (BT_Z_Achse <= -3.2) && (-0.3 <= BT_X_Achse) && (BT_X_Achse<= 0.3)]
  (junction 280) -> Drehen_Links [order 2] : [(Kran_Zyl_Unten || Kran_Zyl_Oben) && Kran_Drehen_Links]
      | {x = x + Kran_Drehen_Schritt;
      | BT_Z_Achse = -3.5*sin(x);
      | BT_X_Achse = 3.5*cos(x);}
  Drehen_Links -> Bauteil_Kran_Rot_Stop [order 2] : [!Kran_Drehen_Links]
  Bauteil_Lager_1_Schieben -> Bauteil_Lager_1_Beginnt : [BT_X_Achse <= -2.7]
  Bauteil_Kran_Rot_Stop -> Drehen_Links [order 1] : [Kran_Drehen_Links]
  Bauteil_Band_Vor -> (junction 135) [order 2]
  Drehen_Links -> (junction 162) [order 4]
  Drehen_Rechts -> Drehen_Links [order 1] : [Kran_Drehen_Links]
  Drehen_Links -> Drehen_Rechts [order 1] : [Kran_Drehen_Rechts]
  Bauteil_Band_Stop -> Bauteil_Band_Vor [order 1] : [Band_Vor]
  Bauteil_Band_Vor -> Bauteil_Band_Stop [order 1] : [!Band_Vor]
  (junction 135) -> Bauteil_Lager_1_Schieben [order 1] : [BT_Z_Achse <= -7.85 && BT_Z_Achse >= -8.65 && Band_Zyl_1_X_Achse >= -0.5]
  Bauteil_Lager_2_Beginnt -> Bauteil_Lager_2_Ende : [BT_X_Achse <= (-6.5 + Lager_2_Status)]
  (junction 280) -> Bauteil_Kran_Rot_Stop [order 3] : [Kran_Zyl_Unten || Kran_Zyl_Oben]
  Drehen_Rechts -> Bauteil_Kran_Rot_Stop [order 2] : [!Kran_Drehen_Rechts]
  Bauteil_Kran_Rot_Stop -> Drehen_Rechts [order 2] : [Kran_Drehen_Rechts]
  Bauteil_Band_Stop -> (junction 135) [order 4]
  (junction 135) -> Bauteil_Lager_2_Schieben [order 3] : [BT_Z_Achse <= -12.05 && BT_Z_Achse >= -12.85 && Band_Zyl_2_X_Achse >= -0.5]
  Bauteil_Band_Zurueck -> (junction 135) [order 2]
  (junction 135) -> Bauteil_Lager_3_Beginnt [order 2] : [BT_Z_Achse <= -14.6]
  Drehen_Rechts -> (junction 162) [order 4]
  Bauteil_Band_Zurueck -> Bauteil_Band_Stop [order 1] : [!Band_Zurueck]
  Bauteil_Band_Stop -> Bauteil_Band_Zurueck [order 2] : [Band_Zurueck]
  Bauteil_Kran_Runterlassen_Und_Drehen_Rechts -> (junction 178) [order 2]
  Bauteil_Kran_Hochheben_Und_Drehen_Links -> (junction 178) [order 2]
  Bauteil_Kran_Hochheben_Und_Drehen_Rechts -> (junction 178) [order 2]
  Bauteil_Kran_Runterlassen_Und_Drehen_Links -> (junction 178) [order 2]
  (junction 280) -> Drehen_Rechts [order 1] : [(Kran_Zyl_Unten || Kran_Zyl_Oben) && Kran_Drehen_Rechts]
      | {x = x - Kran_Drehen_Schritt;
      | BT_Z_Achse = -3.5*sin(x);
      | BT_X_Achse = 3.5*cos(x);}
  (junction 172) -> (junction 280)
  (junction 162) -> Bauteil_Kran_Runterlassen_Und_Drehen_Rechts [order 4] : [Kran_Drehen_Rechts && Kran_Runterlassen]
  (junction 162) -> Bauteil_Kran_Hochheben_Und_Drehen_Rechts [order 2] : [Kran_Drehen_Rechts && Kran_Hochheben]
  (junction 162) -> Bauteil_Kran_Hochheben_Und_Drehen_Links [order 1] : [Kran_Drehen_Links  && Kran_Hochheben]
  (junction 162) -> Bauteil_Kran_Runterlassen_Und_Drehen_Links [order 3] : [Kran_Drehen_Links  && Kran_Runterlassen]
  Bauteil_Lager_2_Schieben -> Bauteil_Lager_2_Beginnt : [BT_X_Achse <= -2.7]
  Bauteil_Kran_Runterlassen_Und_Drehen_Rechts -> (junction 172) [order 1]
  Bauteil_Lager_3_Beginnt -> Bauteil_Lager_3_Ende : [BT_Z_Achse <= (-19.05 + Lager_3_Status)]
  Bauteil_Kran_Hochheben_Und_Drehen_Rechts -> Bauteil_Kran_Runterlassen_Und_Drehen_Rechts [order 3] : [Kran_Drehen_Rechts  && Kran_Runterlassen]
  Bauteil_Kran_Runterlassen_Und_Drehen_Rechts -> Bauteil_Kran_Hochheben_Und_Drehen_Rechts [order 3] : [Kran_Drehen_Rechts  && Kran_Hochheben]
  Bauteil_Kran_Hochheben_Und_Drehen_Rechts -> (junction 172) [order 1]
  Bauteil_Kran_Hochheben_Und_Drehen_Links -> (junction 172) [order 1]
  Bauteil_Kran_Hochheben_Und_Drehen_Links -> Bauteil_Kran_Runterlassen_Und_Drehen_Links [order 3] : [Kran_Drehen_Links  && Kran_Runterlassen]
  Bauteil_Kran_Runterlassen_Und_Drehen_Links -> Bauteil_Kran_Hochheben_Und_Drehen_Links [order 3] : [Kran_Drehen_Links  && Kran_Hochheben]
  Bauteil_Kran_Runterlassen_Und_Drehen_Links -> (junction 172) [order 1]
  data: Achse function_input double; Schrittgroesse function_input double; MaxWert function_input double; Ausgabe function_output double; Achse function_input double; Schrittgroesse function_input double; MinWert function_input double; Ausgabe function_output double; Lager_Status function_input double; Pos_1 function_input double; Pos_2 function_input double; Ausgabe function_output double; Pos_3 function_input double; BT_Y_Achse output double; BT_Lager output double; Kran_Sauger_BT output double; BT_Bereit output double; BT_X_Achse output double; BT_Z_Achse output double; x local double; Lager_X_Achse input; Lager_Ver_Eingefahren input; Lager_Ver_Ausgefahren input; Kran_Stellung_Lager input; Kran_Stellung_Band input; Kran_Stellung_Stempel input; Kran_Zyl_Oben input; Kran_Zyl_Unten input; Kran_Sauger input; Kran_Hochheben input; Kran_Runterlassen input; Kran_Drehen_Links input; Kran_Drehen_Rechts input; Stempel_Halterung_Ausfahren input; Stempel_Halterung_Einfahren input; Band_Vor input; Band_Zurueck input; Band_Zyl_1_X_Achse input; Band_Zyl_2_X_Achse input; BT_Rotation_1 output double; BT_Rotation_2 output double; BT_Rotation_3 output double; BT_Rotation_4 output double; Lager_Ver_Ausfahren input; Lager_Vereinzler_Schritt_Aus input; Kran_Zyl_Schritt_Hoch input; Kran_Zyl_Schritt_Runter input; Kran_Drehen_Schritt input; Stempel_Halterung_Schritt_Aus input; Stempel_Halterung_Schritt_Ein input; Band_Zyl_1_Schritt input; Band_Zyl_2_Schritt input double; Band_Geschwindigkeit input; Bauteil_Fallgeschwindigkeit input double; Lager_1_Status input; Lager_2_Status input; Lager_3_Status input; Naechste_Position local double; BT_1_Bereit input; BT_2_Bereit input; BT_3_Bereit input; BT_4_Bereit input; BT_5_Bereit input; BT_6_Bereit input

== stateflow chart Scenario_13_CoDeSys/Signal Expander/Lager ==
  state r = Continue_Einfahren [function]
    (default) -> (junction 162) : {r=0}
    (junction 162) -> (junction 163) [order 1] : [Vereinzler_Einfahren && !Vereinzler_Ausfahren]
    (junction 163) -> (junction 165) : {r=1}
    (junction 162) -> (junction 164) [order 2]
    (junction 165) -> (junction 164)
  state Schrittgroesse_Ausfahren [function]
    (default) -> (junction 109) : {Schrittgroesse_Ausfahren = (1.65 * Sample_Time)/0.6}
  state Berechne_Naechste_Position_Einfahren [function]
    (default) -> (junction 118) : {Naechste_Position = Vereinzler_X_Achse - Schrittgroesse_Einfahren;}
    (junction 118) -> (junction 120) [order 1] : [Naechste_Position <= -0.65]
    (junction 118) -> (junction 122) [order 2] : {Vereinzler_X_Achse = Naechste_Position;}
    (junction 120) -> (junction 123) : {Vereinzler_X_Achse = -0.65;}
    (junction 123) -> (junction 122)
  state Schrittgroesse_Einfahren [function]
    (default) -> (junction 112) : {Schrittgroesse_Einfahren = (1.65 * Sample_Time)/0.1}
  state Berechne_Naechste_Position_Ausfahren [function]
    (default) -> (junction 208) : {Naechste_Position = Vereinzler_X_Achse + Schrittgroesse_Ausfahren;}
    (junction 208) -> (junction 209) [order 1] : [Naechste_Position >= 1.53]
    (junction 208) -> (junction 210) [order 2] : {Vereinzler_X_Achse = Naechste_Position;}
    (junction 209) -> (junction 211) : {Vereinzler_X_Achse = 1.53;}
    (junction 211) -> (junction 210)
  state r = Stop_Einfahren [function]
    (default) -> (junction 173) : {r=0}
    (junction 173) -> (junction 174) [order 1] : [!Vereinzler_Einfahren || (Vereinzler_Ausfahren && Vereinzler_Einfahren)]
    (junction 174) -> (junction 176) : {r=1}
    (junction 173) -> (junction 175) [order 2]
    (junction 176) -> (junction 175)
  state r = Continue_Ausfahren [function]
    (default) -> (junction 151) : {r=0}
    (junction 151) -> (junction 152) [order 1] : [Vereinzler_Ausfahren && !Vereinzler_Einfahren]
    (junction 152) -> (junction 154) : {r=1}
    (junction 151) -> (junction 153) [order 2]
    (junction 154) -> (junction 153)
  state Vereinzler_Bereit
    entry: Vereinzler_X_Achse = -0.65;
    Vereinzler_Eingefahren = 1;
    exit: Vereinzler_Eingefahren = 0;
  state r = Stop_Ausfahren [function]
    (default) -> (junction 184) : {r=0}
    (junction 184) -> (junction 185) [order 1] : [!Vereinzler_Ausfahren || (Vereinzler_Ausfahren && Vereinzler_Einfahren)]
    (junction 185) -> (junction 187) : {r=1}
    (junction 184) -> (junction 186) [order 2]
    (junction 187) -> (junction 186)
  state Stop1
  state Vereinzler_Ausfahren
    entry: Lager_Ver_Ausfahren = 1;
    during: Vereinzler_X_Achse = Vereinzler_X_Achse + Schrittgroesse_Ausfahren;
    exit: Lager_Ver_Ausfahren = 0;
  state Vereinzler_Ausgefahren_Fertig
    entry: Vereinzler_Ausgefahren = 1;
    Vereinzler_X_Achse = 1.6;
    exit: Vereinzler_Ausgefahren = 0;
  state Vereinzler_Einfahren
    entry: Lager_Ver_Einfahren = 1;
    during: Berechne_Naechste_Position_Einfahren();
    exit: Lager_Ver_Einfahren = 0;
  (default) -> Vereinzler_Bereit : {Schrittgroesse_Ausfahren();
      | Schrittgroesse_Einfahren()}
  Vereinzler_Bereit -> Vereinzler_Ausfahren : [Vereinzler_Ausfahren && !Vereinzler_Einfahren]
  Vereinzler_Einfahren -> Vereinzler_Bereit [order 1] : [Vereinzler_X_Achse <= -0.65]
  Vereinzler_Ausfahren -> Stop1 [order 2] : [!Stop_Einfahren()]
  Stop1 -> Vereinzler_Ausfahren [order 1] : [Continue_Ausfahren()]
  Vereinzler_Ausfahren -> Vereinzler_Ausgefahren_Fertig [order 1] : [Vereinzler_X_Achse >= 1.53]
  Stop1 -> Vereinzler_Einfahren [order 2] : [Continue_Einfahren()]
  Vereinzler_Einfahren -> Stop1 [order 2] : [Stop_Einfahren()]
  Vereinzler_Ausgefahren_Fertig -> Vereinzler_Einfahren : [Vereinzler_Einfahren && !Vereinzler_Ausfahren]
  data: r function_output double; r function_output double; r function_output double; r function_output double; Vereinzler_Einfahren input; Vereinzler_Ausfahren input; Sample_Time input; Vereinzler_X_Achse output double; Vereinzler_Eingefahren output double; Vereinzler_Ausgefahren output double; Lager_Ver_Einfahren output double; Lager_Ver_Ausfahren output double; Schrittgroesse_Ausfahren output double; Schrittgroesse_Einfahren output double; Naechste_Position local double

== stateflow chart Scenario_13_CoDeSys/Signal Expander/Halterung_Stempel ==
  state Halterung_Bereit_Ausgefahren
    entry: Halterung_X_Achse = -1.1;
    Stempel_Halterung_Ausgefahren = 1;
    exit: Stempel_Halterung_Ausgefahren = 0;
  state r = Stop_Einfahren [function]
    (default) -> (junction 63) : {r=0}
    (junction 63) -> (junction 65) [order 1] : [!Halterung_Einfahren || (Halterung_Ausfahren && Halterung_Einfahren)]
    (junction 65) -> (junction 66) : {r=1}
    (junction 63) -> (junction 64) [order 2]
    (junction 66) -> (junction 64)
  state Stop
  state r = Stop_Ausfahren [function]
    (default) -> (junction 77) : {r=0}
    (junction 77) -> (junction 78) [order 1] : [!Halterung_Ausfahren || (Halterung_Ausfahren && Halterung_Einfahren)]
    (junction 78) -> (junction 80) : {r=1}
    (junction 77) -> (junction 79) [order 2]
    (junction 80) -> (junction 79)
  state Halterung_Einfahren
    entry: Stempel_Halterung_Einfahren_FS = 1;
    during: Halterung_X_Achse = Halterung_X_Achse + Schrittgroesse_Einfahren;
    exit: Stempel_Halterung_Einfahren_FS = 0;
  state r = Continue_Einfahren [function]
    (default) -> (junction 88) : {r=0}
    (junction 88) -> (junction 89) [order 1] : [Halterung_Einfahren && !Halterung_Ausfahren]
    (junction 89) -> (junction 91) : {r=1}
    (junction 88) -> (junction 90) [order 2]
    (junction 91) -> (junction 90)
  state Halterung_Eingefahren
    entry: Stempel_Halterung_Eingefahren = 1;
    exit: Stempel_Halterung_Eingefahren = 0;
  state r = Continue_Ausfahren [function]
    (default) -> (junction 110) : {r=0}
    (junction 110) -> (junction 111) [order 1] : [Halterung_Ausfahren && !Halterung_Einfahren]
    (junction 111) -> (junction 113) : {r=1}
    (junction 110) -> (junction 112) [order 2]
    (junction 113) -> (junction 112)
  state Schrittgroesse_Ausfahren [function]
    (default) -> (junction 124) : {Schrittgroesse_Ausfahren = (1.1 * Sample_Time)/0.53}
  state Halterung_ausfahren
    entry: Stempel_Halterung_Ausfahren_FS = 1;
    during: Berechne_Naechste_Position_Ausfahren();
    exit: Stempel_Halterung_Ausfahren_FS = 0;
  state Schrittgroesse_Einfahren [function]
    (default) -> (junction 127) : {Schrittgroesse_Einfahren = (1.1 * Sample_Time)/0.56}
  state Berechne_Naechste_Position_Ausfahren [function]
    (default) -> (junction 133) : {Naechste_Position = Halterung_X_Achse - Schrittgroesse_Ausfahren;}
    (junction 133) -> (junction 134) [order 1] : [Naechste_Position <= -1.1]
    (junction 133) -> (junction 135) [order 2] : {Halterung_X_Achse = Naechste_Position;}
    (junction 134) -> (junction 136) : {Halterung_X_Achse = -1.1;}
    (junction 136) -> (junction 135)
  (default) -> Halterung_Bereit_Ausgefahren : {Schrittgroesse_Ausfahren();
      | Schrittgroesse_Einfahren()}
  Halterung_Bereit_Ausgefahren -> Halterung_Einfahren : [Halterung_Einfahren && !Halterung_Ausfahren]
  Halterung_ausfahren -> Halterung_Bereit_Ausgefahren [order 1] : [Halterung_X_Achse <= -1.1]
  Halterung_Einfahren -> Stop [order 2] : [Stop_Einfahren()]
  Stop -> Halterung_Einfahren [order 2] : [Continue_Einfahren()]
  Halterung_Einfahren -> Halterung_Eingefahren [order 1] : [Halterung_X_Achse >= 0]
  Stop -> Halterung_ausfahren [order 1] : [Continue_Ausfahren()]
  Halterung_ausfahren -> Stop [order 2] : [Stop_Ausfahren()]
  Halterung_Eingefahren -> Halterung_ausfahren : [Halterung_Ausfahren && !Halterung_Einfahren]
  data: r function_output double; r function_output double; r function_output double; r function_output double; Halterung_Ausfahren input; Halterung_Einfahren input; Halterung_X_Achse output double; Stempel_Halterung_Ausgefahren output double; Stempel_Halterung_Eingefahren output double; Stempel_Halterung_Ausfahren_FS output double; Stempel_Halterung_Einfahren_FS output double; Sample_Time input; Schrittgroesse_Ausfahren output double; Schrittgroesse_Einfahren output double; Naechste_Position local double

== stateflow chart Scenario_13_CoDeSys/Signal Expander/Kran ==
  note: 90 Grad = 1.5708
  note: KRan benoetigt fuer 90 Grad 2,6 sek
  state r = Stop_Drehen_Links [function]
    (default) -> (junction 143) : {r=0}
    (junction 143) -> (junction 144) [order 1] : [(!Kran_Drehen_Links || (Kran_Drehen_Links && Kran_Drehen_Rechts)) || (Kran_Stellung >= 3.927)]
    (junction 144) -> (junction 146) : {r=1}
    (junction 143) -> (junction 145) [order 2]
    (junction 146) -> (junction 145)
  state Kran_Drehen_Rechts
    entry: Kran_Drehen_Rechts_FS = 1;
    during: Kran_Stellung = Kran_Stellung - Schrittgroesse_Drehen;
    Kran_Drehwinkel = Kran_Drehwinkel + ((Kran_Drehwinkel_90_Grad * Schrittgroesse_Drehen)/1.5708);
    exit: Kran_Drehen_Rechts_FS = 0;
  state Kran_Drehen_Links
    entry: Kran_Drehen_Links_FS = 1;
    during: Kran_Stellung = Kran_Stellung + Schrittgroesse_Drehen;
    Kran_Drehwinkel = Kran_Drehwinkel - ((Kran_Drehwinkel_90_Grad * Schrittgroesse_Drehen)/1.5708);
    exit: Kran_Drehen_Links_FS = 0;
  state r = Stop_Drehen_Rechts [function]
    (default) -> (junction 187) : {r=0}
    (junction 187) -> (junction 188) [order 1] : [(!Kran_Drehen_Rechts || (Kran_Drehen_Links && Kran_Drehen_Rechts)) || (Kran_Stellung <= -0.7854)]
    (junction 188) -> (junction 190) : {r=1}
    (junction 187) -> (junction 189) [order 2]
    (junction 190) -> (junction 189)
  state r = Continue_Drehen_Links [function]
    (default) -> (junction 200) : {r=0}
    (junction 200) -> (junction 201) [order 1] : [Kran_Drehen_Links && !Kran_Drehen_Rechts && (Kran_Stellung <= 3.927)]
    (junction 201) -> (junction 203) : {r=1}
    (junction 200) -> (junction 202) [order 2]
    (junction 203) -> (junction 202)
  state Kran_Stop
  state r = Continue_Drehen_Rechts [function]
    (default) -> (junction 211) : {r=0}
    (junction 211) -> (junction 212) [order 1] : [!Kran_Drehen_Links && Kran_Drehen_Rechts && (Kran_Stellung >= -0.7854)]
    (junction 212) -> (junction 214) : {r=1}
    (junction 211) -> (junction 213) [order 2]
    (junction 214) -> (junction 213)
  state Schrittgroesse_Drehen [function]
    (default) -> (junction 246) : {Schrittgroesse_Drehen = (1.5708 * Sample_Time)/Kran_Dauer_90_Grad;}
  Kran_Drehen_Links -> Kran_Stop : [Stop_Drehen_Links()]
  Kran_Drehen_Rechts -> Kran_Stop : [Stop_Drehen_Rechts()]
  Kran_Stop -> Kran_Drehen_Rechts [order 2] : [Continue_Drehen_Rechts()]
  Kran_Stop -> Kran_Drehen_Links [order 1] : [Continue_Drehen_Links()]
  (default) -> Kran_Stop : {Schrittgroesse_Drehen();
      | Kran_Drehwinkel = 24300;}
  data: r function_output double; r function_output double; r function_output double; r function_output double; Kran_Drehen_Links input; Kran_Drehen_Rechts input; Kran_Stellung output; Kran_Drehen_Links_FS output; Kran_Drehen_Rechts_FS output; Sample_Time input; Schrittgroesse_Drehen output double; Kran_Drehwinkel output double; Kran_Drehwinkel_90_Grad input double; Kran_Dauer_90_Grad input
